simulink model "traffic_cop"  (Simulink 8.7)
settings: Solver=FixedStepAuto  StartTime=0.0  StopTime=10.0  FixedStep=0.01  RelTol=1e-3
settings Model: Creator=eispin  LastModifiedBy=max
settings DataIOCC: LimitDataPoints=off  SaveFormat=Dataset
settings DebuggingCC: UnderspecifiedInitializationDetection=Simplified  MergeDetectMultiDrivingBlocksExec=error
settings HardwareCC: ProdBitPerPointer=64  ProdLargestAtomicFloat=Float  ProdIntDivRoundTo=Zero  ProdEndianess=LittleEndian  ProdWordSize=64  ProdHWDeviceType=Intel->x86-64 (Windows64)
settings ModelReferenceCC: PropagateSignalLabelsOutOfModel=on
settings ConfigComp: CovModelRefEnable=off

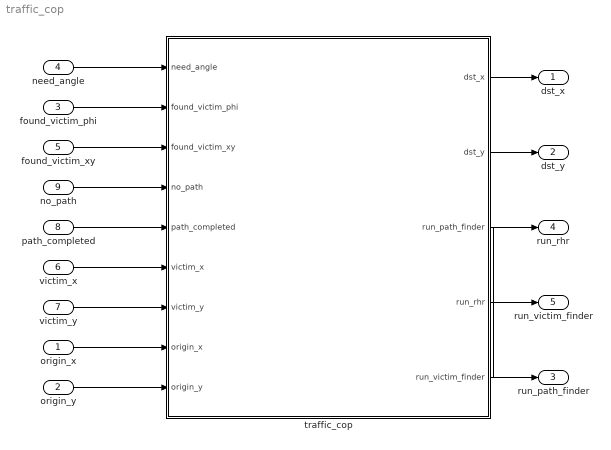
== system traffic_cop ==
  origin_x : Inport
  origin_y : Inport  Port=2
  found_victim_phi : Inport  Port=3
  need_angle : Inport  Port=4
  found_victim_xy : Inport  Port=5
  victim_x : Inport  Port=6
  victim_y : Inport  Port=7
  path_completed : Inport  Port=8
  no_path : Inport  Port=9
  traffic_cop : Stateflow chart  TreatAsAtomicUnit=on
  dst_x : Outport
  dst_y : Outport  Port=2
  run_path_finder : Outport  Port=3
  run_rhr : Outport  Port=4
  run_victim_finder : Outport  Port=5
  wires:
  found_victim_phi/1 -> traffic_cop/2(found_victim_phi)
  need_angle/1 -> traffic_cop/1(need_angle)
  found_victim_xy/1 -> traffic_cop/3(found_victim_xy)
  victim_x/1 -> traffic_cop/6(victim_x)
  victim_y/1 -> traffic_cop/7(victim_y)
  traffic_cop/5(run_victim_finder) -> run_victim_finder/1
  traffic_cop/3(run_path_finder) -> run_path_finder/1
  traffic_cop/4(run_rhr) -> run_rhr/1
  traffic_cop/2(dst_y) -> dst_y/1
  traffic_cop/1(dst_x) -> dst_x/1
  origin_x/1 -> traffic_cop/8(origin_x)
  origin_y/1 -> traffic_cop/9(origin_y)
  path_completed/1 -> traffic_cop/5(path_completed)
  no_path/1 -> traffic_cop/4(no_path)

== stateflow chart traffic_cop ==
  state GetTheLadiesOrGentlemen
    % Done ^.^
    entry:
    run_path_finder = 0;
  state NoPathFound
    % fault tolerance state: no path found but
    % by assumtions there is one -> faulty sensor data -> RHR
    entry:
    run_rhr = 1;
    run_path_finder = 0;
    exit:
    run_rhr = 0;
  state FollowPath
    state RunToVictim
      entry:
      run_rhr = 0;
      run_path_finder = 1;
      dst_x = victim_x;
      dst_y = victim_y;
    state GetOuttaHere
      % not needed, debugging/readability
      entry:
      run_path_finder = 1;
      dst_x = origin_x;
      dst_y = origin_y;
    (default) -> RunToVictim
    RunToVictim -> GetOuttaHere : [path_completed == 1]
  state InitialRHR
    state InitialRHR
      entry:
      run_rhr = 1;
      run_path_finder = 0;
      run_victim_finder = 0;
    state SenseAngle
      entry:
      run_rhr = 0;
      run_victim_finder = 1;
    (default) -> InitialRHR.InitialRHR
    InitialRHR.InitialRHR -> SenseAngle : [need_angle == 1]
    SenseAngle -> InitialRHR.InitialRHR : [found_victim_phi == 1]
  InitialRHR -> FollowPath : [found_victim_xy == 1]
  FollowPath -> NoPathFound : [no_path == 1]
  NoPathFound -> (history) : [after(30, sec)]
  GetOuttaHere -> GetTheLadiesOrGentlemen : [path_completed == 1]
  data: need_angle input double; found_victim_phi input double; found_victim_xy input double; no_path input double; path_completed input double; victim_x input double; victim_y input double; origin_x input double; origin_y input double; dst_x output double; dst_y output double; run_path_finder output double; run_rhr output double; run_victim_finder output double
